simulink model "Vending_Machine"  (R2020b)
settings: Solver=VariableStepAuto  StartTime=0.0  StopTime=200  RelTol=1e-3
settings Model: Creator=vijay jagtap  LastModifiedBy=vijay jagtap

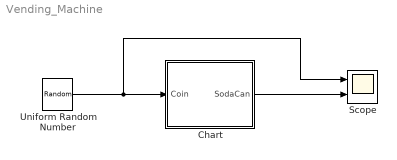
== system Vending_Machine ==
  Chart : Stateflow chart  TreatAsAtomicUnit=on
  Scope : Scope  NumInputPorts=2
  Uniform Random Number : UniformRandomNumber  Minimum=0  Maximum=2  Seed=337  SampleTime=10
  wires:
  Uniform Random Number/1 -> Scope/1, Chart/1(Coin)
  Chart/1(SodaCan) -> Scope/2

== stateflow chart Vending_Machine/Chart ==
  state No_Coin
  state Nickel_Coin
  state Dime_Coin
  (default) -> No_Coin
  Nickel_Coin -> No_Coin [order 1] : [Coin == 2]{SodaCan = 1;}
  Dime_Coin -> No_Coin [order 2] : [Coin == 1]{SodaCan = 1;}
  No_Coin -> Nickel_Coin [order 1] : [Coin == 1]{SodaCan = 0;}
  No_Coin -> Dime_Coin [order 2] : [Coin == 2]{SodaCan = 0;}
  Nickel_Coin -> Dime_Coin [order 2] : [Coin == 1]{SodaCan = 0}
  Dime_Coin -> Nickel_Coin [order 1] : [Coin == 2]{SodaCan = 1}
  data: Coin input; SodaCan output
